simulink model "zeitbereich"  (R2020a)
settings: Solver=VariableStepAuto  StartTime=0.0  StopTime=20  RelTol=1e-3
values from neighbouring files (symbols this model uses):
  A = [0, 1, 0, 0 ... (first row only)    [Aufgabe4.m]    (also in berechnung.m = simplify(subs(A)); reglerInit.m = [0,                1, 0, 0;       -9.81*(1+ml/0.8), 0, 0, 0.; sim_model.m)
  B = [0, -30.49, 0, 30.49]'    [Aufgabe4.m]    (also in berechnung.m = simplify(subs(B)); reglerInit.m = [0; -30.49; 0; 30.49]; sim_model.m)
  C = eye(4)    [Aufgabe4.m]    (also in reglerInit.m = [1, 0, 0, 0;       0, 0, 1, 0]; sim_model.m; zeitbereich_skript.m)
  D = [0;0;0;0]    [Aufgabe4.m]    (also in reglerInit.m = [0; 0]; sim_model.m = [0,0,0,0]'; zeitbereich_skript.m = [0; 0; 0; 0])
  k = place(A, B, poles)    [reglerInit.m]    (also in zeitbereich_skript.m)
  v = -1/(C(2,:)/(A-B*k)*B)    [reglerInit.m]    (also in zeitbereich_skript.m = -1/(C(3,:)/(A-B*k)*B))
  z0 = [0, 0, 0, 0]    [zeitbereich_skript.m]
settings Model: Creator=niko  LastModifiedBy=niko

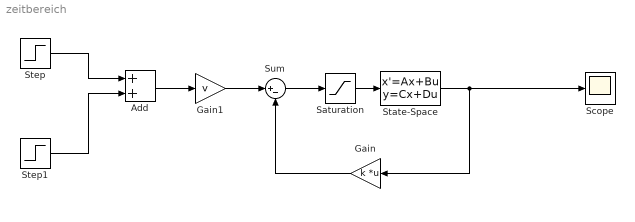
== system zeitbereich ==
  Add : Sum
  Gain : Gain  Gain=k  Multiplication=Matrix(K*u)
  Gain1 : Gain  Gain=v
  Saturation : Saturate  UpperLimit=0.4  LowerLimit=-0.4
  Scope : Scope
  State-Space : StateSpace  A=A  B=B  C=C  D=D  InitialCondition=z0
  Step : Step  SampleTime=0
  Step1 : Step  Time=6  After=-4  SampleTime=0
  Sum : Sum  Inputs=|+-
  wires:
  State-Space/1 -> Scope/1, Gain/1
  Sum/1 -> Saturation/1
  Gain/1 -> Sum/2
  Add/1 -> Gain1/1
  Step/1 -> Add/1
  Step1/1 -> Add/2
  Gain1/1 -> Sum/1
  Saturation/1 -> State-Space/1
